simulink model "continous_nonlinear_model"  (R2024a)
settings: Solver=VariableStepAuto  StartTime=0.0  StopTime=10  RelTol=1e-3
values from neighbouring files (symbols this model uses):
  m = calculate_model(p, T, tau_e)    [init.m]
  omega0 = 20    [init.m]
  reg = syn_regulator(m, 0.1, T)    [init.m]
  T = 0.00064    [init.m]
  tau_e = 0.005    [init.m]
settings Model: Creator=olgatsybina  LastModifiedBy=olgatsybina

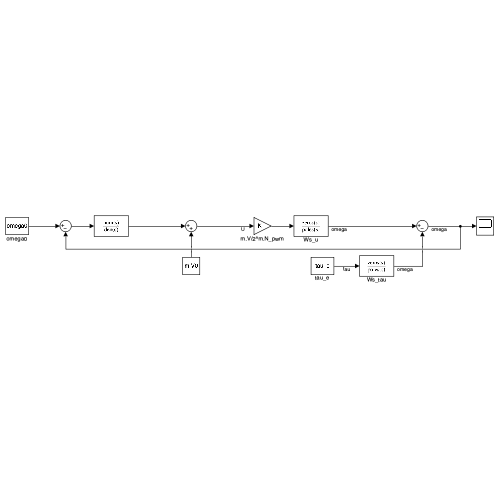
[thumbnail: Simulink's stored preview of the top-level diagram]
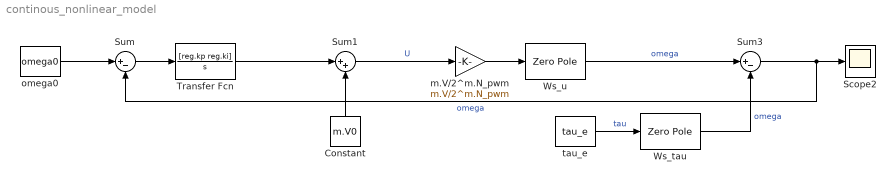
== system continous_nonlinear_model ==
  Constant : Constant  Value=m.V0
  Scope2 : Scope
  Sum : Sum  Inputs=|+-
  Sum1 : Sum  Inputs=|++
  Sum3 : Sum  Inputs=|+-
  Transfer Fcn : TransferFcn  Numerator=[reg.kp reg.ki]  Denominator=[1 0]
  Ws_tau : ZeroPole  Zeros=m.Ws_tau.Z{1}  Poles=m.Ws_tau.P{1}  Gain=m.Ws_tau.K
  Ws_u : ZeroPole  Zeros=m.Ws_u.Z{1}  Poles=m.Ws_u.P{1}  Gain=m.Ws_u.K
  m.V/2^m.N_pwm : Gain  Gain=m.V/2^m.N_pwm
  omega0 : Constant  Value=omega0  SampleTime=T
  tau_e : Constant  Value=tau_e  SampleTime=T
  wires:
  omega0/1 -> Sum/1
  Ws_u/1 -> Sum3/1  "omega"
  Sum3/1 -> Sum/2, Scope2/1  "omega"
  Sum1/1 -> m.V/2^m.N_pwm/1  "U"
  tau_e/1 -> Ws_tau/1  "tau"
  Sum/1 -> Transfer Fcn/1
  Transfer Fcn/1 -> Sum1/1
  m.V/2^m.N_pwm/1 -> Ws_u/1
  Constant/1 -> Sum1/2
  Ws_tau/1 -> Sum3/2  "omega"
